simulink model "Final2"  (R2025b)
settings: Solver=ode23t  StartTime=0.0  StopTime=35  MaxStep=5e-4  RelTol=1e-6  AbsTol=1e-8  EnableMultiTasking=on
values from neighbouring files (symbols this model uses):
  Ad = sysd.A    [MARLUP_FINAL.m]    (also in marlup_params.mat = [1 0 0 0 0 0 0.01 1 0 0 0 0 ... (36 elements, 6x6)]; test.m)
  Bd = sysd.B    [MARLUP_FINAL.m]    (also in marlup_params.mat = [8.07172860911e-06 0.00161434572182 0 0 0 0 0 0 8.0717286091; test.m)
  Cd = sysd.C    [MARLUP_FINAL.m]    (also in marlup_params.mat = [1 0 0 0 0 0 0 1 0 0 0 0 ... (18 elements, 3x6)]; test.m)
  Dd = sysd.D    [MARLUP_FINAL.m]    (also in marlup_params.mat = [0  0  0; 0  0  0; 0  0  0]; test.m)
  F_trim = -W \ c    [MARLUP_FINAL.m]    (also in marlup_identify.m; test.m)
  K = dlqr(Ad, Bd, Q, R)    [MARLUP_FINAL.m]    (also in marlup_params.mat = [223.00056 -1.47048847191e-14 2.18394653467e-12 59.466816 1.; script_will_corregido.m = lqr(A, Bu, Q, R); test.m; tests_will.m = lqr(A, B, Q, R))
  Kr = pinv(Cd * ((eye(6) - Ad + Bd*K) \ Bd))    [MARLUP_FINAL.m]    (also in test.m)
  m = t > tskip & t <= tfit    [marlup_identify.m]    (also in marlup_params.mat = 3; script_will.m = size(B,2); script_will_corregido.m = 3; script_will_old.m = size(B,2))
  N = zeros(size(Gw,2), p)    [script_will.m]    (also in script_will_old.m = zeros(6,3))
  Rn = diag([sigma_ang^2, sigma_ang^2, sigma_z^2])    [MARLUP_FINAL.m]    (also in script_will.m = diag([sigma_ang_sensor^2, sigma_ang_sensor^2, sigma_z_sensor; script_will_old.m = diag([(0.5*pi/180)^2, (0.5*pi/180)^2, (3e-3)^2]); test.m)
  Ts = 0.01    [MARLUP_FINAL.m]    (also in marlup_params.mat; script_will.m; script_will_corregido.m; script_will_old.m)
  Z = squeeze(lg.getElement('Z').Values.Data)    [test.m]
  z0 = 1.571637930257020    (= 1.57163793026)    [MARLUP_FINAL.m]    (also in marlup_identify.m = NaN; test.m = Z(1))
undefined symbols (not defined in the file or in its folder): Discrete, Time, X, Y
libraries: sm_lib x72, nesl_utility x11, ctrlSharedLib x1, dspstat3 x1
(part 4 of 4)

== matlab function Final2/P-M SPECTRUM/P-M SPECTRUM ==
  settings: updateMethod=DISCRETE
  data: t input; heave output; Hs input; Tp input; pitch output; roll output
function [heave, pitch, roll] = fcn(t, Hs, Tp)
%#codegen
% Esta función genera la elevación (heave), y los ángulos de inclinación 
% (pitch y roll) en el origen (0,0) para un oleaje P-M.
%
% Se utiliza t==0 para una inicialización robusta.

% -- Declaración de variables persistentes --
% Estas variables retienen su valor entre llamadas a la función.
persistent Anm fase omega kx ky

% -- Bloque de Inicialización --
% Este código se ejecuta UNA SOLA VEZ, al puro inicio de la simulación (t=0).
if t == 0
    
    % Parámetros fijos de la simulación
    N = 100;         % Número de componentes de frecuencia
    M = 50;          % Número de componentes de dirección
    g = 9.81;        % Aceleración de la gravedad

    % --- PRE-CÁLCULOS (se ejecutan solo una vez) ---
    fp = 1 / Tp;
    f_max = 4 * fp;
    df = f_max / N;
    f = df:df:f_max;
    omega = 2 * pi * f;

    d_theta = 2*pi / M;
    theta = d_theta:d_theta:2*pi;
    
    % Semilla fija: el mismo estado de mar en cada corrida, para poder
    % comparar controladores y reproducir resultados.
    rng(42);

    % Generar fases aleatorias (fijas para toda la simulación)
    fase = 2 * pi * rand(N, M);

    k_o = omega.^2 / g;
    kx = k_o' * cos(theta);
    ky = k_o' * sin(theta);
    
    A_pm = (5/16) * Hs^2 * fp^4;
    S = (A_pm ./ f.^5) .* exp(-1.25 * (fp^4 ./ f.^4));

    s = 10;
    D_theta = (2/pi) * (cos(theta/2)).^(2*s);
    D_theta(theta < -pi/2 | theta > pi/2) = 0;
    
    Anm = sqrt(2 * S' .* D_theta * df * d_theta);
end

% -- CÁLCULOS EN CADA PASO DE TIEMPO --
% Se requiere que las variables persistentes no estén vacías después de t=0
if isempty(Anm)
    % Si la inicialización no ha ocurrido (ej. si la simulación no empezó en t=0),
    % se asignan salidas cero para evitar errores.
    heave = 0;
    pitch = 0;
    roll = 0;
else
    % Cálculos normales para t > 0
    arg = -omega' * t + fase;
    heave = sum(Anm .* cos(arg), 'all');
    d_etadx = sum(Anm .* kx .* sin(arg), 'all');
    d_etady = sum(Anm .* ky .* sin(arg), 'all');
    pitch = atan(d_etadx);
    roll  = atan(d_etady);
end

end
